simulink model "ammclib_amclib_observer_F32_s32k11x"  (Simulink 9.0)
settings: Solver=FixedStepDiscrete  StartTime=0.0  StopTime=10  FixedStep=0.001  RelTol=1e-3  EnableMultiTasking=on
PostLoadFcn:
  | ammclib_amclib_observer_s32k11x_param();
InitFcn:
  | mbd_s32k_consistency_checks(bdroot(gcs));
undefined symbols (not defined in the file or in its folder): LQFP, thumb
libraries: ammclib_bam_s32k11x x17, mbd_s32k1xx_ec_toolbox x2, simulink x1
Description:
  | This model tests the AMMCLIB AMCLIB OBSERVER F32 blocks
  | 
  | Validation:
  | - Run the model in Simulation and check the results
  | - Open Freemaster (ammclib_amclib_observer_F32_s32k11x.pmp) and compare the HW results against the Simulated ones
CloseFcn:
  | clear all;
settings Model: Creator=NXP MBDT Team  LastModifiedBy=nxf35172
settings DataIOCC: ExternalInput=off  InitialState=off  LimitDataPoints=on  SaveOutput=off  SignalLogging=off  SaveTime=off
settings OptimizationCC: DefaultParameterBehavior=Inlined  LifeSpan=1
settings DebuggingCC: SolverPrmCheckMsg=warning  InheritedTsInSrcMsg=none  SingleTaskRateTransMsg=error  IntegerOverflowMsg=none  ParameterPrecisionLossMsg=none  UnconnectedInputMsg=error  UnconnectedOutputMsg=error  UnconnectedLineMsg=error  AllowSymbolicDim=off  UnknownTsInhSupMsg=error  StateNameClashWarn=warning
settings HardwareCC: ProdLargestAtomicInteger=Long  ProdLargestAtomicFloat=Double  ProdEndianess=LittleEndian  ProdHWDeviceType=ARM Compatible->ARM Cortex
settings SFSimCC: MATLABDynamicMemAlloc=off
settings RTWCC: SystemTargetFile=mbd_s32k.tlc  MakeCommand=mbd_s32k_make_rtw COPY_MDLREF_INCLUDES=0  TemplateMakefile=mbd_s32k.tmf  Description=Model Based Design Toolbox S32K14x Code Generation Target
settings CodeAppCC: IgnoreCustomStorageClasses=off
settings STFCustomTargetCC: MultiwordLength=256  CombineOutputUpdateFcns=on  ERTCustomFileBanners=on  SupportContinuousTime=off  SupportNonInlinedSFcns=off  RemoveResetFunc=on  MATLABClassNameForMDSCustomization=Simulink.SoftwareTarget.ERTCustomization  GRTInterface=off  SystemTargetFile=mbd_s32k14.tlc
settings ERTTargetCC: ParMdlRefBuildCompliant=off  CompOptLevelCompliant=off  ConcurrentExecutionCompliant=off  ModelStepFunctionPrototypeControlCompliant=off  CPPClassGenCompliant=off  UseToolchainInfoCompliant=off  InlinedParameterPlacement=NonHierarchical  ERTCustomFileTemplate=example_file_process.tlc  ConvertIfToSwitch=off  SuppressUnreachableDefaultCases=off

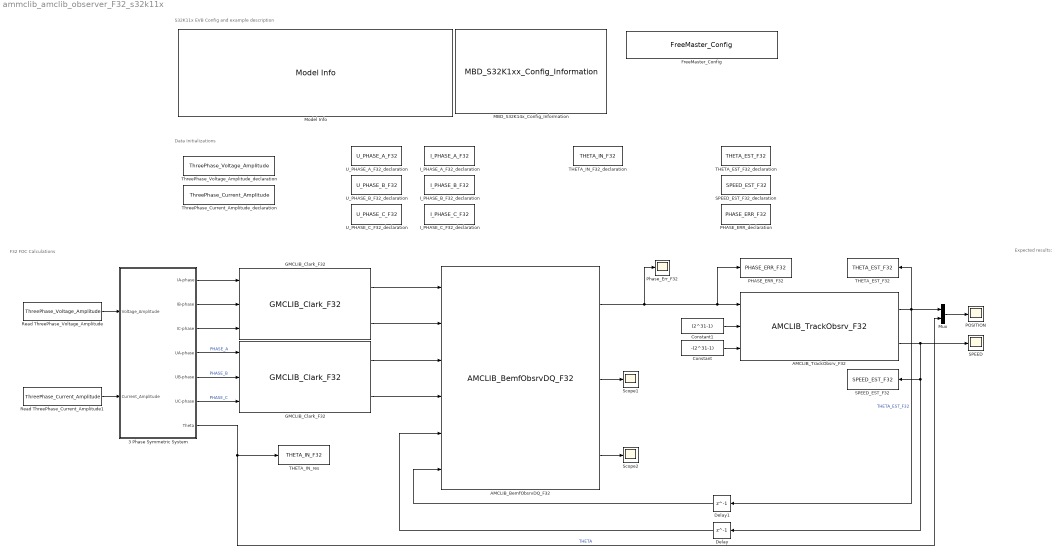
== system ammclib_amclib_observer_F32_s32k11x ==
  note: Expected results:
  note: S32K11x EVB Config and example description
  note: Data Initializations
  note: F32 FOC Calculations
  " Read ThreePhase_Current_Amplitude1" : DataStoreRead  DataStoreName=ThreePhase_Current_Amplitude
  " Read ThreePhase_Voltage_Amplitude" : DataStoreRead  DataStoreName=ThreePhase_Voltage_Amplitude
  3 Phase Symmetric System : Subsystem
  AMCLIB_BemfObsrvDQ_F32 : ammclib_bam_s32k11x/AMCLIB/bam_f32/AMCLIB_BemfObsrvDQ_F32  f32IGain=f32IGain  f32UGain=f32UGain  f32WIGain=f32WIGain  f32EGain=f32EGain  s16Shift=s16Shift  f32CC1sc_D=f32CC1sc_D  f32CC1sc_Q=f32CC1sc_Q  f32CC2sc_D=f32CC2sc_D  f32CC2sc_Q=f32CC2sc_Q  f32UpperLimit_D=f32UpperLimit_D  f32UpperLimit_Q=f32UpperLimit_Q  f32LowerLimit_D=f32LowerLimit_D  f32LowerLimit_Q=f32LowerLimit_Q  u16NShift=u16NShift
  AMCLIB_TrackObsrv_F32 : ammclib_bam_s32k11x/AMCLIB/bam_f32/AMCLIB_TrackObsrv_F32  f32CC1sc=f32CC1sc  f32CC2sc=f32CC2sc  u16NShift=u16NShift  f32C1=f32C1  u16IntegNShift=u16IntegNShift
  Constant : Constant  Value=-(2^31-1)  OutDataTypeStr=Inherit: Inherit via back propagation
  Constant1 : Constant  Value=(2^31-1)  OutDataTypeStr=Inherit: Inherit via back propagation
  Delay : Delay  DelayLength=1  InitialCondition=0
  Delay1 : Delay  DelayLength=1  InitialCondition=0
  FreeMaster_Config : mbd_s32k1xx_ec_toolbox/Utility Blocks/FreeMaster_Config  interface=LPUART0  baudrate=19200  rxd=PTB0: [LPUART0_RX | Receive]  txd=PTB1: [LPUART0_TX | Transmit]  mode=Short Interrupt  isr_prio=1  show_adv_opts=on  use_scope=on  max_scope_vars=8  use_recorder=on  max_rec_vars=8  rec_buff_size=1024  rec_timebase=0 milliseconds  comm_buffer_size_auto=on  comm_buffer_size=255  comm_rqueue_size_default=on  comm_rqueue_size=32
  GMCLIB_Clark_F32 : ammclib_bam_s32k11x/GMCLIB/bam_f32/GMCLIB_Clark_F32
  "GMCLIB_Clark_F32 " : ammclib_bam_s32k11x/GMCLIB/bam_f32/GMCLIB_Clark_F32
  I_PHASE_A_F32_declaration : DataStoreMemory  Priority=2  DataStoreName=I_PHASE_A_F32  ReadBeforeWriteMsg=warning  WriteAfterWriteMsg=warning  WriteAfterReadMsg=warning  ShowAdditionalParam=off  OutDataTypeStr=int32
  I_PHASE_B_F32_declaration : DataStoreMemory  Priority=2  DataStoreName=I_PHASE_B_F32  ReadBeforeWriteMsg=warning  WriteAfterWriteMsg=warning  WriteAfterReadMsg=warning  ShowAdditionalParam=off  OutDataTypeStr=int32
  I_PHASE_C_F32_declaration : DataStoreMemory  Priority=2  DataStoreName=I_PHASE_C_F32  ReadBeforeWriteMsg=warning  WriteAfterWriteMsg=warning  WriteAfterReadMsg=warning  ShowAdditionalParam=off  OutDataTypeStr=int32
  MBD_S32K14x_Config_Information : mbd_s32k1xx_ec_toolbox/MBD_S32K1xx_Config_Information  Priority=0  mbdt_ver=0  disp_str=|  config_params=[]  mcu_target_name=S32K116  mcu_target_package=48-LQFP  mcu_target_sram_size=17KB  mcu_system_clock_freq=40  mcu_xtal_freq=External 40  mcu_steptick_timer=LPIT Channel 0  mcu_steptick_prio=0  ds_import_enable=on  target_compiler=GCC  target_memory=FLASH  gcc_target_compile_opts=-mcpu=cortex-m0plus -mthumb -O1 -g -gstrict-dwarf  gcc_target_assemble_opts=-mcpu=cortex-m0plus -mthumb -g  gcc_target_link_opts=-mcpu=cortex-m0plus -mthumb  gcc_target_default_lcf=on  gcc_target_user_lcf=S32K116_17_flash.ld  ghs_target_compile_opts=-mcpu=cortexm0plus -mthumb -fsoft -Ogeneral -Wundef -Wimplicit-int -Wshadow -Wtrigraphs --no_commons --gnu_asm -gnu99 -gdwarf-2 -G  ghs_target_assemble_opts=-mcpu=cortexm0plus -mthumb -fsoft --gnu_asm  ghs_target_link_opts=-mcpu=cortexm0plus -mthumb -fsoft  ghs_target_default_lcf=off  ghs_target_user_lcf=S32K116_17_flash.ld  iar_target_compile_opts=--thumb -Ol -e --debug --dlib_config normal  iar_target_assemble_opts=--thumb  iar_target_link_opts=--no_exceptions --vfe --inline  iar_target_default_lcf=off  iar_target_user_lcf=S32K116_17_flash.icf  pil_download_enable=off  rbl_download_enable=on  rbl_start_delay=5000000  rbl_download_interface=OpenSDA  rbl_restart_request=off  rbl_com_port=Custom  rbl_com_port_custom=COM1  pil_download_rate=57600  pil_opensda_drive=Custom  pil_opensda_drive_custom=D  pil_uart_instance=0  pil_uart_rx=PTA2: [LPUART0_RX | Receive]  pil_uart_tx=PTA3: [LPUART0_TX | Transmit]  FTM_PWM_PcrCheckEnDis=on  FTM_Input_Edge_Inputs_PcrCheckEnDis=on  FTM_Dual_Edge_Inputs_PcrCheckEnDis=on  FTM_Quadrature_Inputs_PcrCheckEnDis=on  FTM_Hall_Sensor_Inputs_PcrCheckEnDis=on  LPTMR_PcrCheckEnDis=on  PIT_PcrCheckEnDis=on  RTC_PcrCheckEnDis=on  FlexCAN_PcrCheckEnDis=on  LIN_PcrCheckEnDis=on  FlexIO_PcrCheckEnDis=on  LPI2C_PcrCheckEnDis=on  LPSPI_PcrCheckEnDis=on  LPUART_PcrCheckEnDis=on  CMP_PcrCheckEnDis=on  GPIO_OutputPcrCheckEnDis=on  GPIO_InputPcrCheckEnDis=on  SBC_PcrCheckEnDis=on  AMMCLIB_PcrCheckEnDis=on  FM_PcrCheckEnDis=on  Profile_PcrCheckEnDis=on  ConfigParams_PcrCheckEnDis=on  ModelRef_PcrCheckEnDis=on  PDB0_PcrCheckEnDis=on  CSEc_PcrCheckEnDis=on  eDMA_PcrCheckEnDis=on  ADC_PcrCheckEnDis=on  WDOG_PcrCheckEnDis=on
      | Target : S32K142-16KB_SRAM
      | Package : 100-pin
      | System clock : 80 MHz
      | XTAL clock : External 8 MHz
      | Compiler : GCC
      | Target Type : FLASH
      | Download Code after build : (OpenSDA: E)
      | Step Tick Interrupt Priority : 15
  Model Info : simulink/Model-Wide Utilities/Model Info  Frame=off  DisplayStringWithTags=|  HorizontalTextAlignment=Left  LeftAlignmentValue=0.02
      | Model Name: %<ModelName>
      | 
      | Description: %<Description>
  Mux : Mux  Inputs=2
  PHASE_ERR_F32 : DataStoreWrite  DataStoreName=PHASE_ERR_F32
  PHASE_ERR_declaration : DataStoreMemory  Priority=2  DataStoreName=PHASE_ERR_F32  ReadBeforeWriteMsg=warning  WriteAfterWriteMsg=warning  WriteAfterReadMsg=warning  ShowAdditionalParam=off  OutDataTypeStr=int32
  POSITION : Scope
  Phase_Err_F32 : Scope
  SPEED : Scope
  SPEED_EST_F32 : DataStoreWrite  DataStoreName=SPEED_EST_F32
  SPEED_EST_F32_declaration : DataStoreMemory  Priority=2  DataStoreName=SPEED_EST_F32  ReadBeforeWriteMsg=warning  WriteAfterWriteMsg=warning  WriteAfterReadMsg=warning  ShowAdditionalParam=off  OutDataTypeStr=int32
  Scope1 : Scope
  Scope2 : Scope
  THETA_EST_F32 : DataStoreWrite  DataStoreName=THETA_EST_F32
  THETA_EST_F32_declaration : DataStoreMemory  Priority=2  DataStoreName=THETA_EST_F32  ReadBeforeWriteMsg=warning  WriteAfterWriteMsg=warning  WriteAfterReadMsg=warning  ShowAdditionalParam=off  OutDataTypeStr=int32
  THETA_IN_F32_declaration : DataStoreMemory  Priority=2  DataStoreName=THETA_IN_F32  ReadBeforeWriteMsg=warning  WriteAfterWriteMsg=warning  WriteAfterReadMsg=warning  ShowAdditionalParam=off  OutDataTypeStr=int32
  THETA_IN_res : DataStoreWrite  DataStoreName=THETA_IN_F32
  ThreePhase_Current_Amplitude_declaration : DataStoreMemory  Priority=1  DataStoreName=ThreePhase_Current_Amplitude  WriteAfterWriteMsg=warning  WriteAfterReadMsg=warning  InitialValue=0.3*(2^31-1)  ShowAdditionalParam=off  OutMin=-(2^31-1)  OutMax=2^31-1  OutDataTypeStr=int32
  ThreePhase_Voltage_Amplitude_declaration : DataStoreMemory  Priority=1  DataStoreName=ThreePhase_Voltage_Amplitude  WriteAfterWriteMsg=warning  WriteAfterReadMsg=warning  InitialValue=0.61*(2^31-1)  ShowAdditionalParam=off  OutMin=-(2^31-1)  OutMax=2^31-1  OutDataTypeStr=int32
  U_PHASE_A_F32_declaration : DataStoreMemory  Priority=2  DataStoreName=U_PHASE_A_F32  ReadBeforeWriteMsg=warning  WriteAfterWriteMsg=warning  WriteAfterReadMsg=warning  ShowAdditionalParam=off  OutDataTypeStr=int32
  U_PHASE_B_F32_declaration : DataStoreMemory  Priority=2  DataStoreName=U_PHASE_B_F32  ReadBeforeWriteMsg=warning  WriteAfterWriteMsg=warning  WriteAfterReadMsg=warning  ShowAdditionalParam=off  OutDataTypeStr=int32
  U_PHASE_C_F32_declaration : DataStoreMemory  Priority=2  DataStoreName=U_PHASE_C_F32  ReadBeforeWriteMsg=warning  WriteAfterWriteMsg=warning  WriteAfterReadMsg=warning  ShowAdditionalParam=off  OutDataTypeStr=int32
  wires:
  3 Phase Symmetric System/7(Theta) -> Mux/2, THETA_IN_res/1  "THETA"
  " Read ThreePhase_Voltage_Amplitude"/1 -> 3 Phase Symmetric System/1("Voltage_Amplitude ")
  AMCLIB_BemfObsrvDQ_F32/2 -> Scope1/1
  AMCLIB_BemfObsrvDQ_F32/3 -> Scope2/1
  " Read ThreePhase_Current_Amplitude1"/1 -> 3 Phase Symmetric System/2(Current_Amplitude)
  GMCLIB_Clark_F32/1 -> AMCLIB_BemfObsrvDQ_F32/1
  GMCLIB_Clark_F32/2 -> AMCLIB_BemfObsrvDQ_F32/2
  "GMCLIB_Clark_F32 "/1 -> AMCLIB_BemfObsrvDQ_F32/3
  "GMCLIB_Clark_F32 "/2 -> AMCLIB_BemfObsrvDQ_F32/4
  3 Phase Symmetric System/1(IA-phase) -> GMCLIB_Clark_F32/1
  3 Phase Symmetric System/2(IB-phase) -> GMCLIB_Clark_F32/2
  3 Phase Symmetric System/3(IC-phase) -> GMCLIB_Clark_F32/3
  3 Phase Symmetric System/4(UA-phase) -> "GMCLIB_Clark_F32 "/1  "PHASE_A"
  3 Phase Symmetric System/5(UB-phase) -> "GMCLIB_Clark_F32 "/2  "PHASE_B"
  3 Phase Symmetric System/6(UC-phase) -> "GMCLIB_Clark_F32 "/3  "PHASE_C"
  AMCLIB_BemfObsrvDQ_F32/1 -> PHASE_ERR_F32/1, AMCLIB_TrackObsrv_F32/1, Phase_Err_F32/1
  Constant/1 -> AMCLIB_TrackObsrv_F32/3
  Constant1/1 -> AMCLIB_TrackObsrv_F32/2
  AMCLIB_TrackObsrv_F32/1 -> THETA_EST_F32/1, Mux/1, Delay1/1  "THETA_EST_F32"
  AMCLIB_TrackObsrv_F32/2 -> SPEED_EST_F32/1, Delay/1, SPEED/1
  Delay/1 -> AMCLIB_BemfObsrvDQ_F32/5
  Delay1/1 -> AMCLIB_BemfObsrvDQ_F32/6
  Mux/1 -> POSITION/1

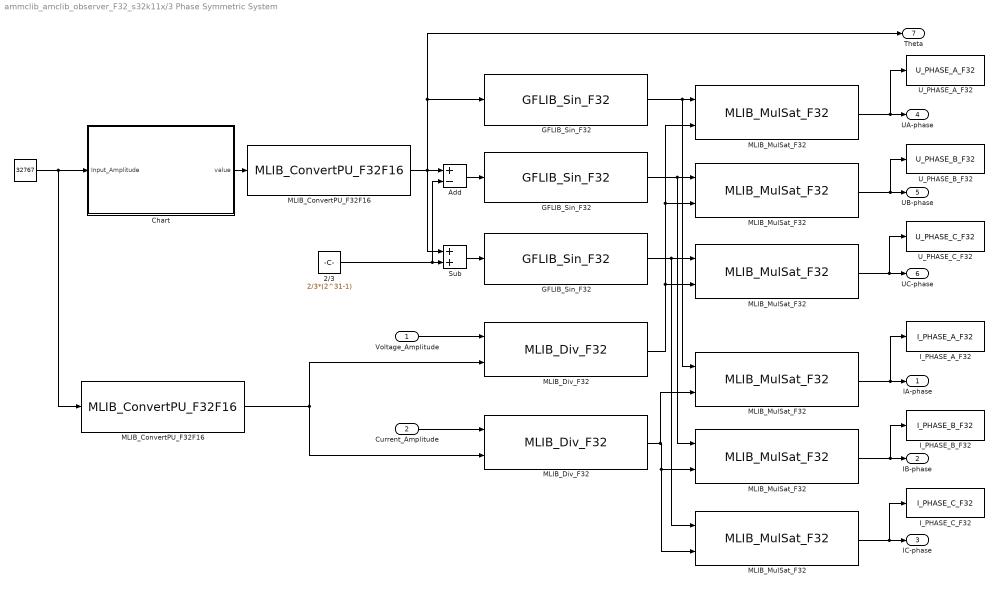
== system ammclib_amclib_observer_F32_s32k11x/3 Phase Symmetric System ==
  "Voltage_Amplitude " : Inport
  Current_Amplitude : Inport  Port=2
  " " : Constant  Value=32767  OutDataTypeStr=int16
  "  MLIB_MulSat_F32  " : ammclib_bam_s32k11x/MLIB/bam_f32/MLIB_MulSat_F32
  " MLIB_MulSat_F32" : ammclib_bam_s32k11x/MLIB/bam_f32/MLIB_MulSat_F32
  " MLIB_MulSat_F32 " : ammclib_bam_s32k11x/MLIB/bam_f32/MLIB_MulSat_F32
  2/3 : Constant  Value=2/3*(2^31-1)  OutDataTypeStr=int32
  Add : Sum  Inputs=+-
  Chart : Stateflow chart  TreatAsAtomicUnit=on
  GFLIB_Sin_F32 : ammclib_bam_s32k11x/GFLIB/bam_f32/GFLIB_Sin_F32
  "GFLIB_Sin_F32 " : ammclib_bam_s32k11x/GFLIB/bam_f32/GFLIB_Sin_F32
  "GFLIB_Sin_F32  " : ammclib_bam_s32k11x/GFLIB/bam_f32/GFLIB_Sin_F32
  I_PHASE_A_F32 : DataStoreWrite  DataStoreName=I_PHASE_A_F32
  I_PHASE_B_F32 : DataStoreWrite  DataStoreName=I_PHASE_B_F32
  I_PHASE_C_F32 : DataStoreWrite  DataStoreName=I_PHASE_C_F32
  MLIB_ConvertPU_F32F16 : ammclib_bam_s32k11x/MLIB/bam_f32/MLIB_ConvertPU_F32F16
  "MLIB_ConvertPU_F32F16    " : ammclib_bam_s32k11x/MLIB/bam_f32/MLIB_ConvertPU_F32F16
  MLIB_Div_F32 : ammclib_bam_s32k11x/MLIB/bam_f32/MLIB_Div_F32
  "MLIB_Div_F32  " : ammclib_bam_s32k11x/MLIB/bam_f32/MLIB_Div_F32
  MLIB_MulSat_F32 : ammclib_bam_s32k11x/MLIB/bam_f32/MLIB_MulSat_F32
  "MLIB_MulSat_F32 " : ammclib_bam_s32k11x/MLIB/bam_f32/MLIB_MulSat_F32
  "MLIB_MulSat_F32  " : ammclib_bam_s32k11x/MLIB/bam_f32/MLIB_MulSat_F32
  Sub : Sum
  U_PHASE_A_F32 : DataStoreWrite  DataStoreName=U_PHASE_A_F32
  U_PHASE_B_F32 : DataStoreWrite  DataStoreName=U_PHASE_B_F32
  U_PHASE_C_F32 : DataStoreWrite  DataStoreName=U_PHASE_C_F32
  IA-phase : Outport
  IB-phase : Outport  Port=2
  IC-phase : Outport  Port=3
  UA-phase : Outport  Port=4
  UB-phase : Outport  Port=5
  UC-phase : Outport  Port=6
  Theta : Outport  Port=7
  wires:
  Chart/1(value) -> MLIB_ConvertPU_F32F16/1
  2/3/1 -> Add/2, Sub/2
  Sub/1 -> "GFLIB_Sin_F32  "/1
  Add/1 -> "GFLIB_Sin_F32 "/1
  "Voltage_Amplitude "/1 -> MLIB_Div_F32/1
  MLIB_Div_F32/1 -> "MLIB_MulSat_F32  "/2, "MLIB_MulSat_F32 "/2, MLIB_MulSat_F32/2
  GFLIB_Sin_F32/1 -> " MLIB_MulSat_F32"/1, MLIB_MulSat_F32/1
  "GFLIB_Sin_F32 "/1 -> " MLIB_MulSat_F32 "/1, "MLIB_MulSat_F32 "/1
  "GFLIB_Sin_F32  "/1 -> "  MLIB_MulSat_F32  "/1, "MLIB_MulSat_F32  "/1
  "MLIB_MulSat_F32 "/1 -> U_PHASE_B_F32/1, UB-phase/1
  "MLIB_MulSat_F32  "/1 -> U_PHASE_C_F32/1, UC-phase/1
  " "/1 -> Chart/1(Input_Amplitude), "MLIB_ConvertPU_F32F16    "/1
  MLIB_MulSat_F32/1 -> U_PHASE_A_F32/1, UA-phase/1
  Current_Amplitude/1 -> "MLIB_Div_F32  "/1
  " MLIB_MulSat_F32 "/1 -> IB-phase/1, I_PHASE_B_F32/1
  "  MLIB_MulSat_F32  "/1 -> IC-phase/1, I_PHASE_C_F32/1
  " MLIB_MulSat_F32"/1 -> IA-phase/1, I_PHASE_A_F32/1
  "MLIB_Div_F32  "/1 -> "  MLIB_MulSat_F32  "/2, " MLIB_MulSat_F32 "/2, " MLIB_MulSat_F32"/2
  MLIB_ConvertPU_F32F16/1 -> Theta/1, GFLIB_Sin_F32/1, Sub/1, Add/1
  "MLIB_ConvertPU_F32F16    "/1 -> MLIB_Div_F32/2, "MLIB_Div_F32  "/2

== stateflow chart 3 Phase Symmetric System/Chart ==
  settings: executeAtInitialization=1
  state A
    du:
    cntr=cntr+25;
    value=cntr;
    ex:
    cntr = -Input_Amplitude;
  (default) -> A : {cntr=0;}
  A -> A : [cntr >= Input_Amplitude]
  data: cntr local int16 =0; value output int16; Input_Amplitude input int16
